simulink model "MAIN_SIMULINK_2023a_yessss"  (R2024b)
settings: Solver=ode45  StartTime=0.0  StopTime=1000  RelTol=1e-7  EnableMultiTasking=on
values from neighbouring files (symbols this model uses):
  f = 1/5    (= 0.2)    [auto_ident_for_app.m]    (also in auto_ident_for_app_v2.m = evalin('base', 'f'); auto_identification.m)
  gp_1 = gp_1/Gain_tec    [auto_ident_for_app.m]    (also in auto_ident_for_app_v2.m = identify(y1, u, t, 1, 0, false, NaN))
  gp_2 = identify(y2, y1, t, 1, 0, true, 5)    [auto_ident_for_app.m]    (also in auto_ident_for_app_v2.m = identify(y2, y1, t, 1, 0, false, NaN))
  gp_3 = identify(y3, y2, t, 1, 0, false, 15)    [auto_ident_for_app.m]    (also in auto_ident_for_app_v2.m = identify(y3, y2, t, 1, 0, false, NaN))
undefined symbols (not defined in the file or in its folder): A, A_2, B, B_2, C, C_2, consigne_finale, consigne_init, consigne_step_time, D, D_2, dac_bit, DFz, filt_pwm, freq_pwm, gain1, gain2, gain3, gain_amp, gpp_1, gpp_2, gpp_3, kc, offset1, offset2, offset3, pert_finale, pert_init, pert_step_time, R_fixe, sat_c, sat_f, T_init, tec_gains, tec_tension, Tiz, Z_T3
libraries: simulink_extras x6, simulink x1
settings Model: Creator=LiberT  LastModifiedBy=Mathieu Bouchard
settings SolverCC: AlgebraicLoopSolver=TrustRegion
settings DataIOCC: LimitDataPoints=on  SaveFormat=Array  SignalLoggingSaveFormat=ModelDataLogs  ReturnWorkspaceOutputs=off
settings OptimizationCC: BlockReduction=off  BooleanDataType=off  ExpressionDepthLimit=2147483647  InitFltsAndDblsToZero=on  LifeSpan=inf
settings DebuggingCC: SaveWithParameterizedLinksMsg=none  UnderspecifiedInitializationDetection=Classic  MergeDetectMultiDrivingBlocksExec=none  SignalResolutionControl=TryResolveAllWithWarning  MultiTaskDSMMsg=warning  MultiTaskCondExecSysMsg=none  FcnCallInpInsideContextMsg=warning  UnconnectedInputMsg=warning  UnconnectedOutputMsg=warning  UnconnectedLineMsg=warning  StateNameClashWarn=warning  SFUnexpectedBacktrackingDiag=warning  SFNoUnconditionalDefaultTransitionDiag=warning  SFExecutionAtInitializationDiag=none  ArithmeticOperatorsInVariantConditions=warning
settings HardwareCC: ProdBitPerPointer=32  ProdBitPerSizeT=32  ProdBitPerPtrDiffT=32  ProdLargestAtomicFloat=None  ProdIntDivRoundTo=Undefined  ProdEndianess=Unspecified  ProdWordSize=32  ProdHWDeviceType=32-bit Generic  TargetUnknown=on
settings ModelReferenceCC: EnableRefExpFcnMdlSchedulingChecks=on  PropagateSignalLabelsOutOfModel=off
settings SFSimCC: SimUseLocalCustomCode=off  LegacyBehaviorForPersistentVarInContinuousTime=on  CustomCodeUndefinedFunction=UseInterfaceOnly
settings RTWCC: RTWUseLocalCustomCode=off  GPUComputeCapability=3.5
settings CodeAppCC: StateflowObjectComments=on
settings GRTTargetCC: TargetFcnLib=ansi_tfl_tmw.mat  TargetLangStandard=C89/C90 (ANSI)  ModelReferenceCompliant=off  CompOptLevelCompliant=off  CombineOutputUpdateFcns=off  MatFileLogging=off  GRTInterface=on
settings ConfigComp: CovMetricSettings=dw  CovSaveCumulativeToWorkspaceVar=on  CovSaveSingleToWorkspaceVar=on  CovExternalEMLEnable=off

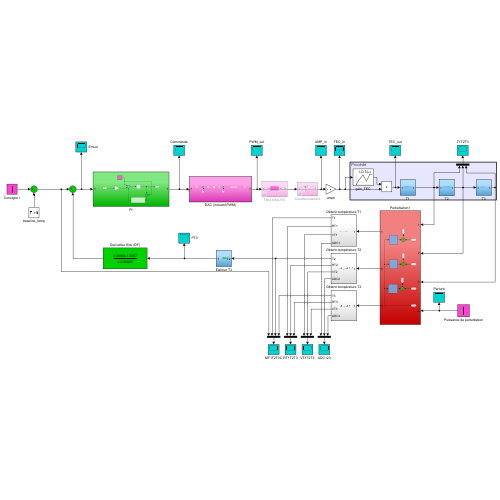
[thumbnail: Simulink's stored preview of the top-level diagram]
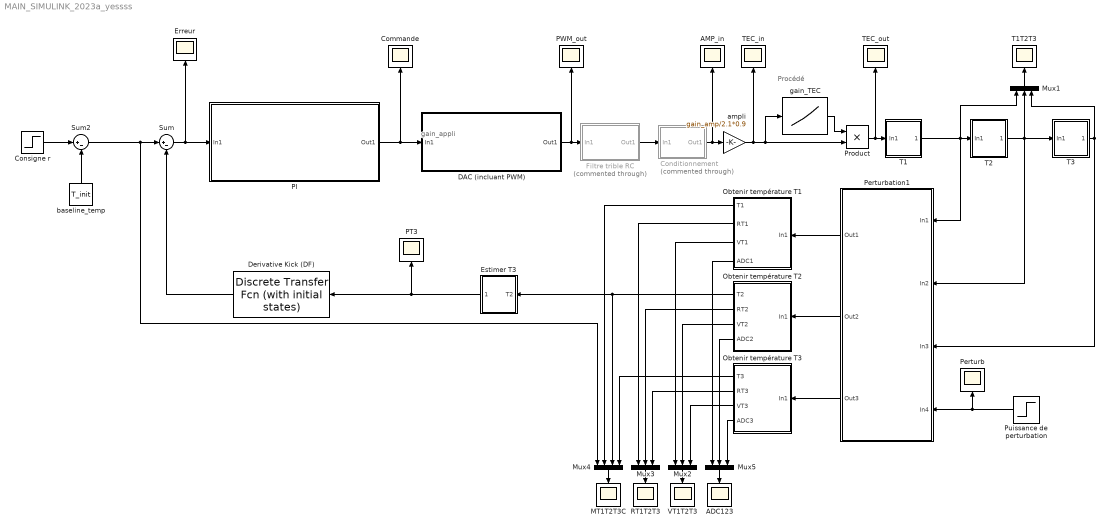
== system MAIN_SIMULINK_2023a_yessss ==
  note: gain_appli
  note: Procédé
  ADC123 : Scope
  AMP_in : Scope
  Commande : Scope
  Conditionnement : Subsystem  Commented=through
  Consigne r : Step  Time=consigne_step_time  Before=consigne_init  After=consigne_finale  SampleTime=0
  DAC (incluant PWM) : Subsystem
  Derivative Kick (DF) : simulink_extras/Additional Discrete/Discrete Transfer Fcn (with initial states)  N=DFz.Numerator{1}  D=DFz.Denominator{1}  X0=[0]  TS=1/f
  Erreur : Scope
  Estimer T3 : Subsystem
  Filtre trible RC : Subsystem  Commented=through
  MT1T2T3C : Scope
  Mux{1..3,5} (4 alike) : Mux  Inputs=3
  Mux4 : Mux
  Obtenir température T1 : Subsystem
  Obtenir température T2 : Subsystem
  Obtenir température T3 : Subsystem
  PI : Subsystem
  PT3 : Scope
  PWM_out : Scope
  Perturb : Scope
  Perturbation1 : Subsystem
  Product : Product
  Puissance de perturbation : Step  Time=pert_step_time  Before=pert_init  After=pert_finale  SampleTime=1/f
  RT1T2T3 : Scope
  Sum : Sum  Inputs=|+-  InputSameDT=on  SaturateOnIntegerOverflow=on  OutDataTypeStr=Inherit: Same as first input
  Sum2 : Sum  Inputs=|+-  InputSameDT=on  SaturateOnIntegerOverflow=on  OutDataTypeStr=Inherit: Same as first input
  T1 : Subsystem
  T1T2T3 : Scope
  T2 : Subsystem
  T3 : Subsystem
  TEC_in : Scope
  TEC_out : Scope
  VT1T2T3 : Scope
  ampli : Gain  Gain=gain_amp/2.1*0.9
  baseline_temp : Constant  Value=T_init
  gain_TEC : Lookup_n-D  NumberOfTableDimensions=1  BreakpointsForDimension1=tec_tension  Table=tec_gains  InternalRulePriority=Speed  RndMeth=Simplest
  wires:
  Consigne r/1 -> Sum2/1
  baseline_temp/1 -> Sum2/2
  PI/1(Out1) -> DAC (incluant PWM)/1(In1), Commande/1
  Sum/1 -> PI/1(In1), Erreur/1
  DAC (incluant PWM)/1(Out1) -> Filtre trible RC/1(In1), PWM_out/1
  Filtre trible RC/1(Out1) -> Conditionnement/1(In1)
  Derivative Kick (DF)/1 -> Sum/2
  T2/1(Out1) -> Perturbation1/2(In2), T3/1(In1), Mux1/2
  T1/1(Out1) -> Perturbation1/1(In1), Mux1/1, T2/1(In1)
  Estimer T3/1(Out1) -> PT3/1, Derivative Kick (DF)/1
  T3/1(Out1) -> Perturbation1/3(In3), Mux1/3
  gain_TEC/1 -> Product/1
  Product/1 -> TEC_out/1, T1/1(In1)
  Perturbation1/2(Out2) -> Obtenir température T2/1(In1)
  Conditionnement/1(Out1) -> AMP_in/1, ampli/1
  Perturbation1/3(Out3) -> Obtenir température T3/1(In1)
  Mux1/1 -> T1T2T3/1
  Perturbation1/1(Out1) -> Obtenir température T1/1(In1)
  Obtenir température T2/1(T2) -> Estimer T3/1(T2), Mux4/3
  Obtenir température T3/3(VT3) -> Mux2/3
  Obtenir température T2/3(VT2) -> Mux2/2
  Obtenir température T1/3(VT1) -> Mux2/1
  Mux2/1 -> VT1T2T3/1
  Mux3/1 -> RT1T2T3/1
  Obtenir température T3/2(RT3) -> Mux3/3
  Obtenir température T2/2(RT2) -> Mux3/2
  Obtenir température T1/2(RT1) -> Mux3/1
  Mux4/1 -> MT1T2T3C/1
  Sum2/1 -> Mux4/1, Sum/1
  Obtenir température T3/1(T3) -> Mux4/4
  Obtenir température T1/1(T1) -> Mux4/2
  Mux5/1 -> ADC123/1
  Obtenir température T3/4(ADC3) -> Mux5/3
  Obtenir température T2/4(ADC2) -> Mux5/2
  Obtenir température T1/4(ADC1) -> Mux5/1
  ampli/1 -> TEC_in/1, Product/2, gain_TEC/1
  Puissance de perturbation/1 -> Perturbation1/4(In4), Perturb/1

== system MAIN_SIMULINK_2023a_yessss/Conditionnement ==
  In1 : Inport
  Offset2 : Constant  Value=-2.5
  Sum10 : Sum  Inputs=|++  InputSameDT=on  SaturateOnIntegerOverflow=on  OutDataTypeStr=Inherit: Same as first input
  gain_condi : Gain  Gain=1/2.5
  Out1 : Outport
  wires:
  Sum10/1 -> gain_condi/1
  gain_condi/1 -> Out1/1
  Offset2/1 -> Sum10/2
  In1/1 -> Sum10/1

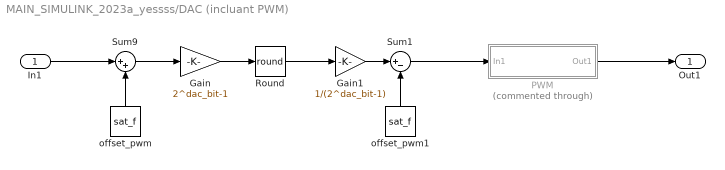
== system MAIN_SIMULINK_2023a_yessss/DAC (incluant PWM) ==
  In1 : Inport
  Gain : Gain  Gain=2^dac_bit-1
  Gain1 : Gain  Gain=1/(2^dac_bit-1)
  PWM : Subsystem  Commented=through
  Round : Rounding  Operator=round
  Sum1 : Sum  Inputs=|+-  InputSameDT=on  SaturateOnIntegerOverflow=on  OutDataTypeStr=Inherit: Same as first input
  Sum9 : Sum  Inputs=|++  InputSameDT=on  SaturateOnIntegerOverflow=on  OutDataTypeStr=Inherit: Same as first input
  offset_pwm : Constant  Value=sat_f
  offset_pwm1 : Constant  Value=sat_f
  Out1 : Outport
  wires:
  Gain/1 -> Round/1
  offset_pwm/1 -> Sum9/2
  In1/1 -> Sum9/1
  Sum9/1 -> Gain/1
  Round/1 -> Gain1/1
  Sum1/1 -> PWM/1(In1)
  offset_pwm1/1 -> Sum1/2
  Gain1/1 -> Sum1/1
  PWM/1(Out1) -> Out1/1

== system MAIN_SIMULINK_2023a_yessss/Estimer T3 ==
  T2 : Inport
  Delay : Delay  DelayLength=Z_T3.IODelay  InitialCondition=0
  Derivative Kick (DF) : simulink_extras/Additional Discrete/Discrete Transfer Fcn (with initial states)  N=Z_T3.num{1}  D=Z_T3.den{1}  X0=[0]  TS=1/f
  Out1 : Outport
  wires:
  T2/1 -> Delay/1
  Delay/1 -> Derivative Kick (DF)/1
  Derivative Kick (DF)/1 -> Out1/1

== system MAIN_SIMULINK_2023a_yessss/Filtre trible RC ==
  In1 : Inport
  Filtre triple RC : TransferFcn  Numerator=filt_pwm.Numerator{1}  Denominator=filt_pwm.Denominator{1}
  Out1 : Outport
  wires:
  Filtre triple RC/1 -> Out1/1
  In1/1 -> Filtre triple RC/1

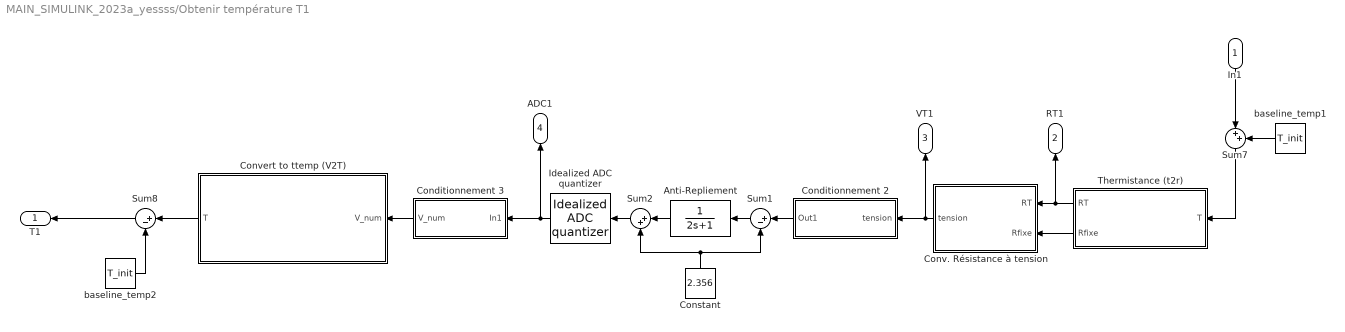
== system MAIN_SIMULINK_2023a_yessss/Obtenir température T1 ==
  In1 : Inport
  Anti-Repliement : TransferFcn  Denominator=[2 1]  ParameterTunability=Optimized
  Conditionnement 2 : Subsystem
  Conditionnement 3 : Subsystem
  Constant : Constant  Value=2.356
  Conv. Résistance à tension : MATLAB Function  TreatAsAtomicUnit=on
  Convert to ttemp (V2T) : Subsystem
  Idealized ADC quantizer : simulink_extras/Additional Discrete/Idealized ADC quantizer  NumberOfConverterBits=adc_bit  Vmin=0  Vmax=5  OutputDataType=double  OutputNegativeValues=off
  Sum1 : Sum  Inputs=|+-  InputSameDT=on  SaturateOnIntegerOverflow=on  OutDataTypeStr=Inherit: Same as first input
  Sum2 : Sum  Inputs=|++  InputSameDT=on  SaturateOnIntegerOverflow=on  OutDataTypeStr=Inherit: Same as first input
  Sum7 : Sum  Inputs=|++  InputSameDT=on  SaturateOnIntegerOverflow=on  OutDataTypeStr=Inherit: Same as first input
  Sum8 : Sum  Inputs=|+-  InputSameDT=on  SaturateOnIntegerOverflow=on  OutDataTypeStr=Inherit: Same as first input
  Thermistance (t2r) : Subsystem
  baseline_temp1 : Constant  Value=T_init
  baseline_temp2 : Constant  Value=T_init
  T1 : Outport
  RT1 : Outport  Port=2
  VT1 : Outport  Port=3
  ADC1 : Outport  Port=4
  wires:
  baseline_temp2/1 -> Sum8/2
  Thermistance (t2r)/1(RT) -> RT1/1, Conv. Résistance à tension/1(RT)
  Sum7/1 -> Thermistance (t2r)/1(T)
  Convert to ttemp (V2T)/1(T) -> Sum8/1
  baseline_temp1/1 -> Sum7/2
  In1/1 -> Sum7/1
  Sum8/1 -> T1/1
  Idealized ADC quantizer/1 -> ADC1/1, Conditionnement 3/1(In1)
  Conv. Résistance à tension/1(tension) -> VT1/1, Conditionnement 2/1(tension)
  Conditionnement 2/1(Out1) -> Sum1/1
  Thermistance (t2r)/2(Rfixe) -> Conv. Résistance à tension/2(Rfixe)
  Conditionnement 3/1(V_num) -> Convert to ttemp (V2T)/1(V_num)
  Sum1/1 -> Anti-Repliement/1
  Sum2/1 -> Idealized ADC quantizer/1
  Anti-Repliement/1 -> Sum2/1
  Constant/1 -> Sum1/2, Sum2/2

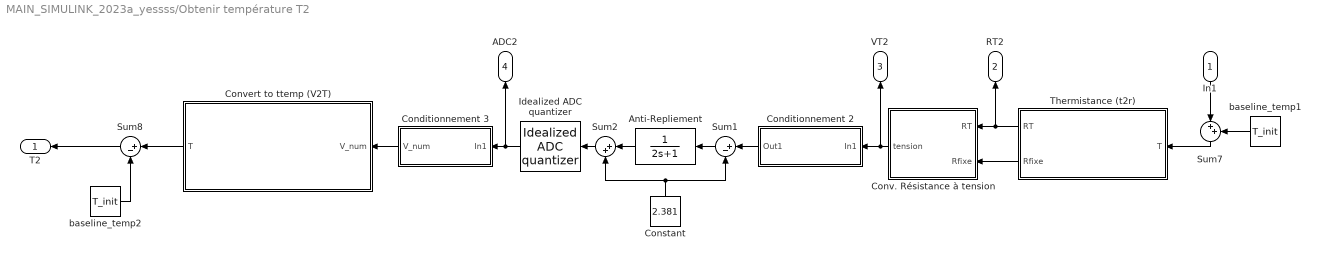
== system MAIN_SIMULINK_2023a_yessss/Obtenir température T2 ==
  In1 : Inport
  Anti-Repliement : TransferFcn  Denominator=[2 1]  ParameterTunability=Optimized
  Conditionnement 2 : Subsystem
  Conditionnement 3 : Subsystem
  Constant : Constant  Value=2.381
  Conv. Résistance à tension : MATLAB Function  TreatAsAtomicUnit=on
  Convert to ttemp (V2T) : Subsystem
  Idealized ADC quantizer : simulink_extras/Additional Discrete/Idealized ADC quantizer  NumberOfConverterBits=adc_bit  Vmin=0  Vmax=5  OutputDataType=double  OutputNegativeValues=off
  Sum1 : Sum  Inputs=|+-  InputSameDT=on  SaturateOnIntegerOverflow=on  OutDataTypeStr=Inherit: Same as first input
  Sum2 : Sum  Inputs=|++  InputSameDT=on  SaturateOnIntegerOverflow=on  OutDataTypeStr=Inherit: Same as first input
  Sum7 : Sum  Inputs=|++  InputSameDT=on  SaturateOnIntegerOverflow=on  OutDataTypeStr=Inherit: Same as first input
  Sum8 : Sum  Inputs=|+-  InputSameDT=on  SaturateOnIntegerOverflow=on  OutDataTypeStr=Inherit: Same as first input
  Thermistance (t2r) : Subsystem
  baseline_temp1 : Constant  Value=T_init
  baseline_temp2 : Constant  Value=T_init
  T2 : Outport
  RT2 : Outport  Port=2
  VT2 : Outport  Port=3
  ADC2 : Outport  Port=4
  wires:
  baseline_temp2/1 -> Sum8/2
  Idealized ADC quantizer/1 -> ADC2/1, Conditionnement 3/1(In1)
  Thermistance (t2r)/1(RT) -> Conv. Résistance à tension/1(RT), RT2/1
  Sum7/1 -> Thermistance (t2r)/1(T)
  baseline_temp1/1 -> Sum7/2
  In1/1 -> Sum7/1
  Conv. Résistance à tension/1(tension) -> Conditionnement 2/1(In1), VT2/1
  Thermistance (t2r)/2(Rfixe) -> Conv. Résistance à tension/2(Rfixe)
  Sum8/1 -> T2/1
  Convert to ttemp (V2T)/1(T) -> Sum8/1
  Conditionnement 3/1(V_num) -> Convert to ttemp (V2T)/1(V_num)
  Constant/1 -> Sum1/2, Sum2/2
  Sum1/1 -> Anti-Repliement/1
  Anti-Repliement/1 -> Sum2/1
  Conditionnement 2/1(Out1) -> Sum1/1
  Sum2/1 -> Idealized ADC quantizer/1

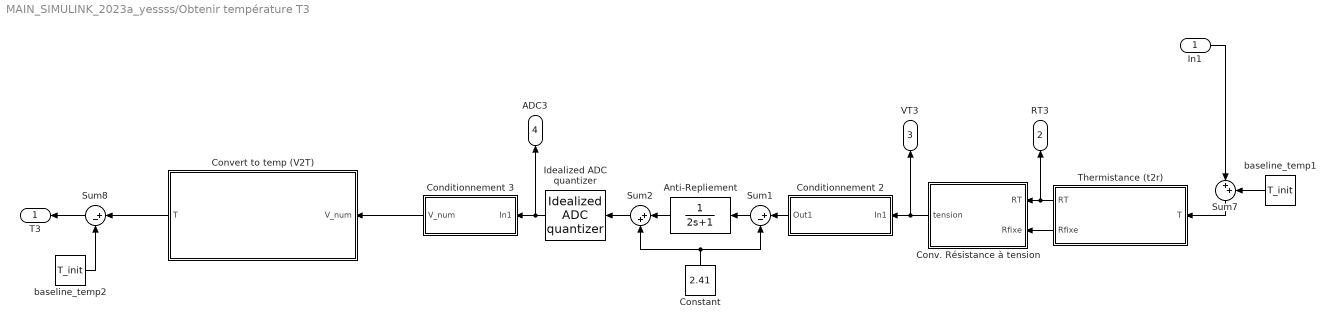
== system MAIN_SIMULINK_2023a_yessss/Obtenir température T3 ==
  In1 : Inport
  Anti-Repliement : TransferFcn  Denominator=[2 1]  ParameterTunability=Optimized
  Conditionnement 2 : Subsystem
  Conditionnement 3 : Subsystem
  Constant : Constant  Value=2.41
  Conv. Résistance à tension : MATLAB Function  TreatAsAtomicUnit=on
  Convert to temp (V2T) : Subsystem
  Idealized ADC quantizer : simulink_extras/Additional Discrete/Idealized ADC quantizer  NumberOfConverterBits=adc_bit  Vmin=0  Vmax=5  OutputDataType=double  OutputNegativeValues=off
  Sum1 : Sum  Inputs=|+-  InputSameDT=on  SaturateOnIntegerOverflow=on  OutDataTypeStr=Inherit: Same as first input
  Sum2 : Sum  Inputs=|++  InputSameDT=on  SaturateOnIntegerOverflow=on  OutDataTypeStr=Inherit: Same as first input
  Sum7 : Sum  Inputs=|++  InputSameDT=on  SaturateOnIntegerOverflow=on  OutDataTypeStr=Inherit: Same as first input
  Sum8 : Sum  Inputs=|+-  InputSameDT=on  SaturateOnIntegerOverflow=on  OutDataTypeStr=Inherit: Same as first input
  Thermistance (t2r) : Subsystem
  baseline_temp1 : Constant  Value=T_init
  baseline_temp2 : Constant  Value=T_init
  T3 : Outport
  RT3 : Outport  Port=2
  VT3 : Outport  Port=3
  ADC3 : Outport  Port=4
  wires:
  baseline_temp2/1 -> Sum8/2
  Idealized ADC quantizer/1 -> ADC3/1, Conditionnement 3/1(In1)
  Thermistance (t2r)/1(RT) -> RT3/1, Conv. Résistance à tension/1(RT)
  Sum7/1 -> Thermistance (t2r)/1(T)
  baseline_temp1/1 -> Sum7/2
  In1/1 -> Sum7/1
  Conv. Résistance à tension/1(tension) -> VT3/1, Conditionnement 2/1(In1)
  Thermistance (t2r)/2(Rfixe) -> Conv. Résistance à tension/2(Rfixe)
  Sum8/1 -> T3/1
  Conditionnement 3/1(V_num) -> Convert to temp (V2T)/1(V_num)
  Convert to temp (V2T)/1(T) -> Sum8/1
  Constant/1 -> Sum1/2, Sum2/2
  Anti-Repliement/1 -> Sum2/1
  Sum1/1 -> Anti-Repliement/1
  Sum2/1 -> Idealized ADC quantizer/1
  Conditionnement 2/1(Out1) -> Sum1/1

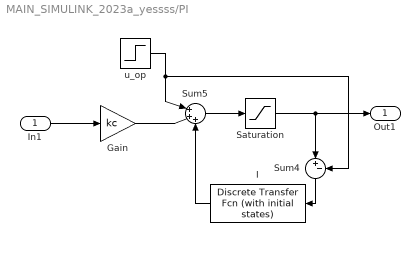
== system MAIN_SIMULINK_2023a_yessss/PI ==
  In1 : Inport
  Gain : Gain  Gain=kc
  I : simulink_extras/Additional Discrete/Discrete Transfer Fcn (with initial states)  N=Tiz.Numerator{1}  D=Tiz.Denominator{1}  X0=[0]  TS=1/f
  Saturation : Saturate  UpperLimit=sat_c  LowerLimit=sat_f
  Sum4 : Sum  Inputs=|+-  InputSameDT=on  SaturateOnIntegerOverflow=on  OutDataTypeStr=Inherit: Same as first input
  Sum5 : Sum  Inputs=|+++  InputSameDT=on  SaturateOnIntegerOverflow=on  OutDataTypeStr=Inherit: Same as first input
  u_op : Step  Time=0  Before=0.001  After=0.001  SampleTime=0
  Out1 : Outport
  wires:
  u_op/1 -> Sum5/1, Sum4/2
  I/1 -> Sum5/3
  Saturation/1 -> Out1/1, Sum4/1
  Sum5/1 -> Saturation/1
  Sum4/1 -> I/1
  In1/1 -> Gain/1
  Gain/1 -> Sum5/2

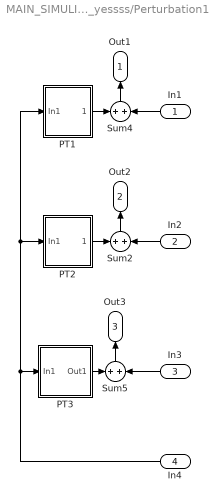
== system MAIN_SIMULINK_2023a_yessss/Perturbation1 ==
  In1 : Inport
  In2 : Inport  Port=2
  In3 : Inport  Port=3
  In4 : Inport  Port=4
  PT1 : Subsystem
  PT2 : Subsystem
  PT3 : Subsystem
  Sum2 : Sum  Inputs=+|+  InputSameDT=on  SaturateOnIntegerOverflow=on  OutDataTypeStr=Inherit: Same as first input
  Sum4 : Sum  Inputs=+|+  InputSameDT=on  SaturateOnIntegerOverflow=on  OutDataTypeStr=Inherit: Same as first input
  Sum5 : Sum  Inputs=+|+  InputSameDT=on  SaturateOnIntegerOverflow=on  OutDataTypeStr=Inherit: Same as first input
  Out1 : Outport
  Out2 : Outport  Port=2
  Out3 : Outport  Port=3
  wires:
  In4/1 -> PT2/1(In1), PT1/1(In1), PT3/1(In1)
  Sum5/1 -> Out3/1
  Sum4/1 -> Out1/1
  In3/1 -> Sum5/2
  PT3/1(Out1) -> Sum5/1
  PT1/1(Out1) -> Sum4/1
  In1/1 -> Sum4/2
  PT2/1(Out1) -> Sum2/1
  Sum2/1 -> Out2/1
  In2/1 -> Sum2/2

== system MAIN_SIMULINK_2023a_yessss/T1 ==
  In1 : Inport
  Dynamique2 : TransferFcn  Numerator=gp_1.num{1}  Denominator=gp_1.den{1}
  Retard2 : TransportDelay  DelayTime=gp_1.IODelay  BufferSize=20000
  Out1 : Outport
  wires:
  In1/1 -> Dynamique2/1
  Dynamique2/1 -> Retard2/1
  Retard2/1 -> Out1/1

== system MAIN_SIMULINK_2023a_yessss/T2 ==
  In1 : Inport
  Dynamique1 : TransferFcn  Numerator=gp_2.num{1}  Denominator=gp_2.den{1}
  Retard2 : TransportDelay  DelayTime=gp_2.IODelay  BufferSize=20000
  Out1 : Outport
  wires:
  Dynamique1/1 -> Out1/1
  In1/1 -> Retard2/1
  Retard2/1 -> Dynamique1/1

== system MAIN_SIMULINK_2023a_yessss/T3 ==
  In1 : Inport
  Dynamique3 : TransferFcn  Numerator=gp_3.Numerator{1}  Denominator=gp_3.Denominator{1}
  Retard3 : TransportDelay  DelayTime=gp_3.IODelay  BufferSize=20000
  Out1 : Outport
  wires:
  Dynamique3/1 -> Out1/1
  Retard3/1 -> Dynamique3/1
  In1/1 -> Retard3/1

== system MAIN_SIMULINK_2023a_yessss/DAC (incluant PWM)/PWM ==
  In1 : Inport
  PWM : simulink/Discontinuities/PWM  DisableCoverage=on  Period=1/freq_pwm  InitialDelay=0  DisallowZeroDutyCycle=off  RunAtFixedTimeIntervals=off  SampleTime=0.1
  Sum9 : Sum  Inputs=|++  InputSameDT=on  SaturateOnIntegerOverflow=on  OutDataTypeStr=Inherit: Same as first input
  gain_pwm1 : Gain  Gain=0.5
  gain_pwm2 : Gain  Gain=5
  offset_pwm : Constant
  Out1 : Outport
  wires:
  gain_pwm2/1 -> Out1/1
  PWM/1 -> gain_pwm2/1
  gain_pwm1/1 -> PWM/1
  Sum9/1 -> gain_pwm1/1
  offset_pwm/1 -> Sum9/2
  In1/1 -> Sum9/1

== system MAIN_SIMULINK_2023a_yessss/Obtenir température T1/Conditionnement 2 ==
  note: Fait un offset et un gain
  tension : Inport
  Sum1 : Sum  Inputs=|+-  InputSameDT=on  SaturateOnIntegerOverflow=on  OutDataTypeStr=Inherit: Same as first input
  gain_in : Gain  Gain=gain1
  offset : Constant  Value=offset1
  Out1 : Outport
  wires:
  gain_in/1 -> Out1/1
  offset/1 -> Sum1/2
  Sum1/1 -> gain_in/1
  tension/1 -> Sum1/1

== system MAIN_SIMULINK_2023a_yessss/Obtenir température T1/Conditionnement 3 ==
  In1 : Inport
  "  " : Gain  Gain=1/gain1
  "   " : Gain  Gain=5/1023
  Sum6 : Sum  Inputs=|++  InputSameDT=on  SaturateOnIntegerOverflow=on  OutDataTypeStr=Inherit: Same as first input
  offset1 : Constant  Value=offset1
  V_num : Outport
  wires:
  "  "/1 -> "   "/1
  offset1/1 -> Sum6/2
  "   "/1 -> Sum6/1
  Sum6/1 -> V_num/1
  In1/1 -> "  "/1

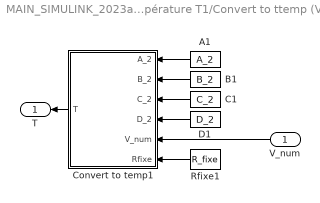
== system MAIN_SIMULINK_2023a_yessss/Obtenir température T1/Convert to ttemp (V2T) ==
  V_num : Inport
  A1 : Constant  Value=A_2
  B1 : Constant  Value=B_2
  C1 : Constant  Value=C_2
  Convert to temp1 : MATLAB Function  TreatAsAtomicUnit=on
  D1 : Constant  Value=D_2
  Rfixe1 : Constant  Value=R_fixe
  T : Outport
  wires:
  B1/1 -> Convert to temp1/2(B_2)
  V_num/1 -> Convert to temp1/5(V_num)
  A1/1 -> Convert to temp1/1(A_2)
  Rfixe1/1 -> Convert to temp1/6(Rfixe)
  C1/1 -> Convert to temp1/3(C_2)
  Convert to temp1/1(T) -> T/1
  D1/1 -> Convert to temp1/4(D_2)

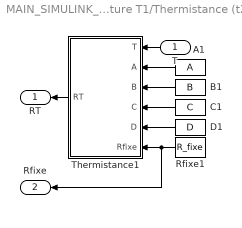
== system MAIN_SIMULINK_2023a_yessss/Obtenir température T1/Thermistance (t2r) ==
  T : Inport
  A1 : Constant  Value=A
  B1 : Constant  Value=B
  C1 : Constant  Value=C
  D1 : Constant  Value=D
  Rfixe1 : Constant  Value=R_fixe
  Thermistance1 : MATLAB Function  TreatAsAtomicUnit=on
  RT : Outport
  Rfixe : Outport  Port=2
  wires:
  Thermistance1/1(RT) -> RT/1
  B1/1 -> Thermistance1/3(B)
  C1/1 -> Thermistance1/4(C)
  T/1 -> Thermistance1/1(T)
  D1/1 -> Thermistance1/5(D)
  Rfixe1/1 -> Rfixe/1, Thermistance1/6(Rfixe)
  A1/1 -> Thermistance1/2(A)

== system MAIN_SIMULINK_2023a_yessss/Obtenir température T2/Conditionnement 2 ==
  note: Fait un offset et un gain
  In1 : Inport
  Sum1 : Sum  Inputs=|+-  InputSameDT=on  SaturateOnIntegerOverflow=on  OutDataTypeStr=Inherit: Same as first input
  gain_in : Gain  Gain=gain2
  offset : Constant  Value=offset2
  Out1 : Outport
  wires:
  gain_in/1 -> Out1/1
  offset/1 -> Sum1/2
  Sum1/1 -> gain_in/1
  In1/1 -> Sum1/1

== system MAIN_SIMULINK_2023a_yessss/Obtenir température T2/Conditionnement 3 ==
  In1 : Inport
  "  " : Gain  Gain=1/gain2
  "   " : Gain  Gain=5/1023
  Sum6 : Sum  Inputs=|++  InputSameDT=on  SaturateOnIntegerOverflow=on  OutDataTypeStr=Inherit: Same as first input
  offset1 : Constant  Value=offset2
  V_num : Outport
  wires:
  "  "/1 -> "   "/1
  offset1/1 -> Sum6/2
  "   "/1 -> Sum6/1
  Sum6/1 -> V_num/1
  In1/1 -> "  "/1

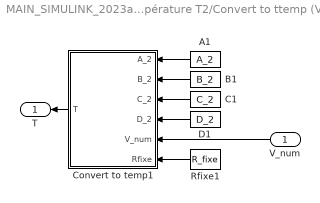
== system MAIN_SIMULINK_2023a_yessss/Obtenir température T2/Convert to ttemp (V2T) ==
  V_num : Inport
  A1 : Constant  Value=A_2
  B1 : Constant  Value=B_2
  C1 : Constant  Value=C_2
  Convert to temp1 : MATLAB Function  TreatAsAtomicUnit=on
  D1 : Constant  Value=D_2
  Rfixe1 : Constant  Value=R_fixe
  T : Outport
  wires:
  D1/1 -> Convert to temp1/4(D_2)
  Convert to temp1/1(T) -> T/1
  C1/1 -> Convert to temp1/3(C_2)
  Rfixe1/1 -> Convert to temp1/6(Rfixe)
  A1/1 -> Convert to temp1/1(A_2)
  V_num/1 -> Convert to temp1/5(V_num)
  B1/1 -> Convert to temp1/2(B_2)

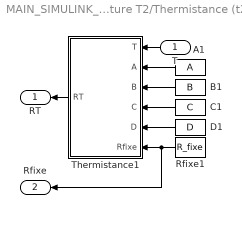
== system MAIN_SIMULINK_2023a_yessss/Obtenir température T2/Thermistance (t2r) ==
  T : Inport
  A1 : Constant  Value=A
  B1 : Constant  Value=B
  C1 : Constant  Value=C
  D1 : Constant  Value=D
  Rfixe1 : Constant  Value=R_fixe
  Thermistance1 : MATLAB Function  TreatAsAtomicUnit=on
  RT : Outport
  Rfixe : Outport  Port=2
  wires:
  Thermistance1/1(RT) -> RT/1
  B1/1 -> Thermistance1/3(B)
  C1/1 -> Thermistance1/4(C)
  T/1 -> Thermistance1/1(T)
  D1/1 -> Thermistance1/5(D)
  Rfixe1/1 -> Rfixe/1, Thermistance1/6(Rfixe)
  A1/1 -> Thermistance1/2(A)

== system MAIN_SIMULINK_2023a_yessss/Obtenir température T3/Conditionnement 2 ==
  note: Fait un offset et un gain
  In1 : Inport
  Sum1 : Sum  Inputs=|+-  InputSameDT=on  SaturateOnIntegerOverflow=on  OutDataTypeStr=Inherit: Same as first input
  gain_in : Gain  Gain=gain3
  offset : Constant  Value=offset3
  Out1 : Outport
  wires:
  gain_in/1 -> Out1/1
  offset/1 -> Sum1/2
  Sum1/1 -> gain_in/1
  In1/1 -> Sum1/1

== system MAIN_SIMULINK_2023a_yessss/Obtenir température T3/Conditionnement 3 ==
  In1 : Inport
  "  " : Gain  Gain=1/gain3
  "   " : Gain  Gain=5/1023
  Sum6 : Sum  Inputs=|++  InputSameDT=on  SaturateOnIntegerOverflow=on  OutDataTypeStr=Inherit: Same as first input
  offset1 : Constant  Value=offset3
  V_num : Outport
  wires:
  "  "/1 -> "   "/1
  offset1/1 -> Sum6/2
  "   "/1 -> Sum6/1
  Sum6/1 -> V_num/1
  In1/1 -> "  "/1

== system MAIN_SIMULINK_2023a_yessss/Obtenir température T3/Convert to temp (V2T) ==
  V_num : Inport
  A1 : Constant  Value=A_2
  B1 : Constant  Value=B_2
  C1 : Constant  Value=C_2
  Convert to temp1 : MATLAB Function  TreatAsAtomicUnit=on
  D1 : Constant  Value=D_2
  Rfixe1 : Constant  Value=R_fixe
  T : Outport
  wires:
  D1/1 -> Convert to temp1/4(D_2)
  Convert to temp1/1(T) -> T/1
  C1/1 -> Convert to temp1/3(C_2)
  Rfixe1/1 -> Convert to temp1/6(Rfixe)
  A1/1 -> Convert to temp1/1(A_2)
  V_num/1 -> Convert to temp1/5(V_num)
  B1/1 -> Convert to temp1/2(B_2)

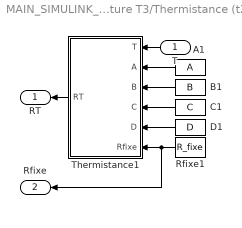
== system MAIN_SIMULINK_2023a_yessss/Obtenir température T3/Thermistance (t2r) ==
  T : Inport
  A1 : Constant  Value=A
  B1 : Constant  Value=B
  C1 : Constant  Value=C
  D1 : Constant  Value=D
  Rfixe1 : Constant  Value=R_fixe
  Thermistance1 : MATLAB Function  TreatAsAtomicUnit=on
  RT : Outport
  Rfixe : Outport  Port=2
  wires:
  Thermistance1/1(RT) -> RT/1
  B1/1 -> Thermistance1/3(B)
  C1/1 -> Thermistance1/4(C)
  T/1 -> Thermistance1/1(T)
  D1/1 -> Thermistance1/5(D)
  Rfixe1/1 -> Rfixe/1, Thermistance1/6(Rfixe)
  A1/1 -> Thermistance1/2(A)

== system MAIN_SIMULINK_2023a_yessss/Perturbation1/PT1 ==
  In1 : Inport
  Dynamique1 : TransferFcn  Numerator=gpp_1.num{1}  Denominator=gpp_1.den{1}
  Retard2 : TransportDelay  DelayTime=gpp_1.IODelay  BufferSize=5000
  Out1 : Outport
  wires:
  Dynamique1/1 -> Retard2/1
  In1/1 -> Dynamique1/1
  Retard2/1 -> Out1/1

== system MAIN_SIMULINK_2023a_yessss/Perturbation1/PT2 ==
  In1 : Inport
  Dynamique1 : TransferFcn  Numerator=gpp_2.num{1}  Denominator=gpp_2.den{1}
  Retard2 : TransportDelay  DelayTime=gpp_2.IODelay  BufferSize=5000
  Out1 : Outport
  wires:
  In1/1 -> Dynamique1/1
  Dynamique1/1 -> Retard2/1
  Retard2/1 -> Out1/1

== system MAIN_SIMULINK_2023a_yessss/Perturbation1/PT3 ==
  In1 : Inport
  Dynamique1 : TransferFcn  Numerator=gpp_3.num{1}  Denominator=gpp_3.den{1}
  Retard2 : TransportDelay  DelayTime=gpp_3.IODelay  BufferSize=5000
  Out1 : Outport
  wires:
  Dynamique1/1 -> Retard2/1
  Retard2/1 -> Out1/1
  In1/1 -> Dynamique1/1

== matlab function MAIN_SIMULINK_2023a_yessss/Obtenir température T1/Conv. Résistance à tension ==
  data: RT input; tension output; Rfixe input
function tension = r2v(RT, Rfixe)
% Définition des coefficients
tension = 5*(RT)/(RT+Rfixe);
end

== matlab function MAIN_SIMULINK_2023a_yessss/Obtenir température T2/Thermistance (t2r)/Thermistance1 ==
  data: T input; RT output; A input; B input; C input; D input; Rfixe input
function RT = t2r(T, A, B, C, D, Rfixe)
% Calcul de la résistance
RT = Rfixe * exp(A + B/(T+273.15) + C/(T+273.15)^2 + D/(T+273.15)^3);
end

== matlab function MAIN_SIMULINK_2023a_yessss/Obtenir température T1/Convert to ttemp (V2T)/Convert to temp1 ==
  data: A_2 input; B_2 input; C_2 input; D_2 input; V_num input; Rfixe input; T output
function T = v2t(A_2, B_2, C_2, D_2, V_num, Rfixe)
RT = Rfixe / (5.0 /V_num - 1.0);
lnR = log(RT / Rfixe);   
T = (1.0 / (A_2 + B_2 * lnR + C_2 * lnR * lnR + D_2 * lnR * lnR * lnR)) - 273.15;
end

== matlab function MAIN_SIMULINK_2023a_yessss/Obtenir température T2/Conv. Résistance à tension ==
  data: RT input; tension output; Rfixe input
function tension = r2v(RT, Rfixe)
% Définition des coefficients
tension = 5*(RT)/(RT+Rfixe);
end

== matlab function MAIN_SIMULINK_2023a_yessss/Obtenir température T3/Convert to temp (V2T)/Convert to temp1 ==
  data: A_2 input; B_2 input; C_2 input; D_2 input; V_num input; Rfixe input; T output
function T = v2t(A_2, B_2, C_2, D_2, V_num, Rfixe)
RT = Rfixe / (5.0 /V_num - 1.0);
lnR = log(RT / Rfixe);   
T = (1.0 / (A_2 + B_2 * lnR + C_2 * lnR * lnR + D_2 * lnR * lnR * lnR)) - 273.15;
end

== matlab function MAIN_SIMULINK_2023a_yessss/Obtenir température T3/Thermistance (t2r)/Thermistance1 ==
  data: T input; RT output; A input; B input; C input; D input; Rfixe input
function RT = t2r(T, A, B, C, D, Rfixe)
% Calcul de la résistance
RT = Rfixe * exp(A + B/(T+273.15) + C/(T+273.15)^2 + D/(T+273.15)^3);
end

== matlab function MAIN_SIMULINK_2023a_yessss/Obtenir température T3/Conv. Résistance à tension ==
  data: RT input; tension output; Rfixe input
function tension = r2v(RT, Rfixe)
tension = 5*(RT)/(RT+Rfixe);
end

== matlab function MAIN_SIMULINK_2023a_yessss/Obtenir température T1/Thermistance (t2r)/Thermistance1 ==
  data: T input; RT output; A input; B input; C input; D input; Rfixe input
function RT = t2r(T, A, B, C, D, Rfixe)
% Calcul de la résistance
RT = Rfixe * exp(A + B/(T+273.15) + C/(T+273.15)^2 + D/(T+273.15)^3);
end

== matlab function MAIN_SIMULINK_2023a_yessss/Obtenir température T2/Convert to ttemp (V2T)/Convert to temp1 ==
  data: A_2 input; B_2 input; C_2 input; D_2 input; V_num input; Rfixe input; T output
function T = v2t(A_2, B_2, C_2, D_2, V_num, Rfixe)
RT = Rfixe / (5.0 /V_num - 1.0);
lnR = log(RT / Rfixe);   
T = (1.0 / (A_2 + B_2 * lnR + C_2 * lnR * lnR + D_2 * lnR * lnR * lnR)) - 273.15;
end
